simulink model "speed"  (R2015b)
settings: Solver=VariableStepAuto  StartTime=0.0  StopTime=20  RelTol=1e-3
settings Model: Creator=朱明菲  LastModifiedBy=朱明菲

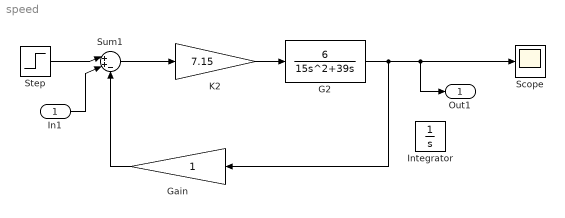
== system speed ==
  In1 : Inport
  G2 : TransferFcn  Numerator=[6]  Denominator=[15 39 0]
  Gain : Gain
  Integrator : Integrator
  K2 : Gain  Gain=7.15
  Scope : Scope
  Step : Step  SampleTime=0
  Sum1 : Sum  Inputs=|++-
  Out1 : Outport
  wires:
  K2/1 -> G2/1
  Step/1 -> Sum1/1
  Sum1/1 -> K2/1
  G2/1 -> Gain/1, Out1/1, Scope/1
  In1/1 -> Sum1/2
  Gain/1 -> Sum1/3
